simulink model "geniusController"  (R2017a)
settings: Solver=VariableStepAuto  StartTime=0.0  StopTime=inf  RelTol=1e-3
libraries: vrlib x1, sldrtlib x1
settings Model: Creator=laure  LastModifiedBy=laure

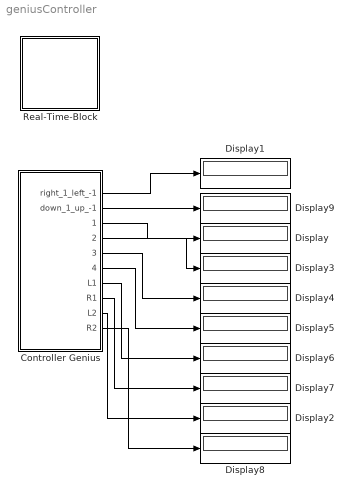
== system geniusController ==
  Controller Genius : Subsystem
  Display{,1..9} (10 alike) : Display
  Real-Time-Block : Subsystem
  wires:
  Controller Genius/3(1) -> Display/1
  Controller Genius/1(right_1_left_-1) -> Display1/1
  Controller Genius/9(L2) -> Display2/1
  Controller Genius/10(R2) -> Display8/1
  Controller Genius/8(R1) -> Display7/1
  Controller Genius/7(L1) -> Display6/1
  Controller Genius/6(4) -> Display5/1
  Controller Genius/5(3) -> Display4/1
  Controller Genius/4(2) -> Display3/1
  Controller Genius/2(down_1_up_-1) -> Display9/1

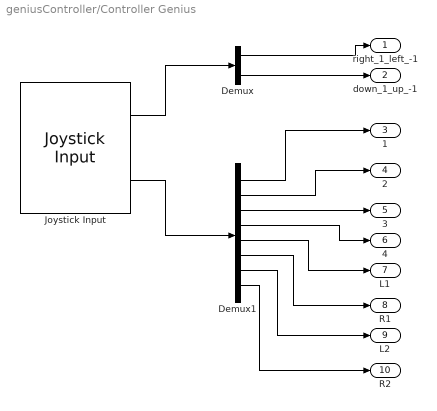
== system geniusController/Controller Genius ==
  Demux : Demux  Outputs=2
  Demux1 : Demux  Outputs=8
  Joystick Input : vrlib/Joystick Input  joyid=1  adjustports=on  forcefeed=off
      settings: SourceProductBaseCode=VR
  right_1_left_-1 : Outport
  down_1_up_-1 : Outport  Port=2
  1 : Outport  Port=3
  2 : Outport  Port=4
  3 : Outport  Port=5
  4 : Outport  Port=6
  L1 : Outport  Port=7
  R1 : Outport  Port=8
  L2 : Outport  Port=9
  R2 : Outport  Port=10
  wires:
  Joystick Input/1 -> Demux/1
  Joystick Input/2 -> Demux1/1
  Demux1/1 -> 1/1
  Demux1/2 -> 2/1
  Demux1/8 -> R2/1
  Demux1/5 -> L1/1
  Demux1/4 -> 4/1
  Demux/1 -> right_1_left_-1/1
  Demux1/6 -> R1/1
  Demux1/7 -> L2/1
  Demux1/3 -> 3/1
  Demux/2 -> down_1_up_-1/1

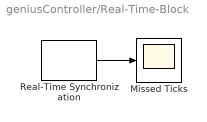
== system geniusController/Real-Time-Block ==
  Missed Ticks : Scope
  Real-Time Synchronization : sldrtlib/Real-Time Synchronization  SampleTime=0.1  MaxMissedTicks=10  ShowMissedTicks=on  YieldWhenWaiting=off
  wires:
  Real-Time Synchronization/1 -> Missed Ticks/1
